simulink model "particle_sim"  (Simulink 8.7)
settings: Solver=ode3  StartTime=0.0  StopTime=inf  RelTol=1e-3
undefined symbols (not defined in the file or in its folder): ProperlyScaledOppositeMover
settings Model: Creator=KAMAK  LastModifiedBy=rcooper
settings DataIOCC: SignalLoggingSaveFormat=ModelDataLogs
settings OptimizationCC: ExpressionDepthLimit=2147483647
settings DebuggingCC: SolverPrmCheckMsg=warning  FcnCallInpInsideContextMsg=UseLocalSettings  StateNameClashWarn=warning
settings GRTTargetCC: CombineOutputUpdateFcns=off  GRTInterface=on

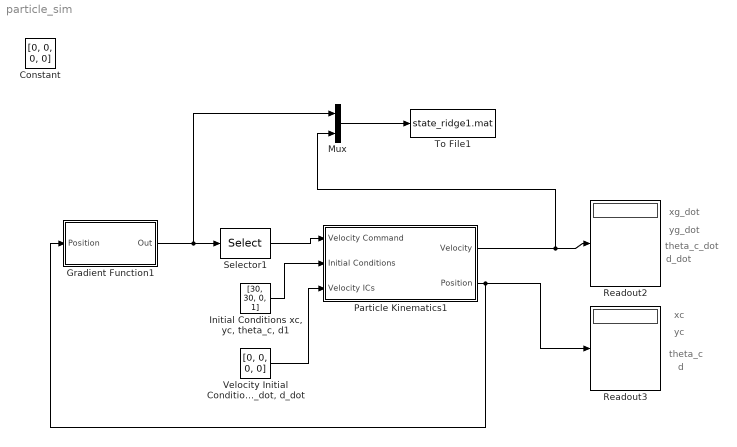
== system particle_sim ==
  note: xg_dot
  note: yg_dot
  note: theta_c_dot
  note: d_dot
  note: xc
  note: yc
  note: theta_c
  note: d
  Gradient Function1 : Subsystem
  "Initial Conditions xc, yc, theta_c, d1" : Constant  Value=[30, 30, 0, 1]  OutDataTypeStr=double
  Mux : Mux  Inputs=2
  Particle Kinematics1 : Subsystem
  Readout2 : Display
  Readout3 : Display
  Selector1 : Selector  InputPortWidth=24  IndexOptions=Index vector (dialog)  Indices=[1 2 3 4]  OutputSizes=1
  To File1 : ToFile  Filename=state_ridge1.mat  MatrixName=data  SaveFormat=Timeseries
  "Velocity Initial Conditions xg_dot, yg_dot, theta_c_dot, d_dot" : Constant  Value=[0, 0, 0, 0]
  Constant : Constant  IOType=siggen  Value=[0, 0, 0, 0]  VectorParams1D=off
  wires:
  "Initial Conditions xc, yc, theta_c, d1"/1 -> Particle Kinematics1/2(Initial Conditions)
  Gradient Function1/1(Out) -> Mux/1, Selector1/1
  Particle Kinematics1/2(Position) -> Gradient Function1/1(Position), Readout3/1
  Particle Kinematics1/1(Velocity) -> Mux/2, Readout2/1
  Selector1/1 -> Particle Kinematics1/1(Velocity Command)
  "Velocity Initial Conditions xg_dot, yg_dot, theta_c_dot, d_dot"/1 -> Particle Kinematics1/3(Velocity ICs)
  Mux/1 -> To File1/1

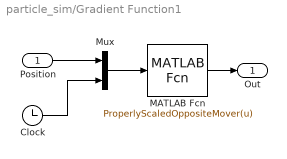
== system particle_sim/Gradient Function1 ==
  Position : Inport
  Clock : Clock
  MATLAB Fcn : MATLABFcn  MATLABFcn=ProperlyScaledOppositeMover(u)  OutputDimensions=24  Output1D=off
  Mux : Mux  Inputs=2
  Out : Outport
  wires:
  MATLAB Fcn/1 -> Out/1
  Clock/1 -> Mux/2
  Position/1 -> Mux/1
  Mux/1 -> MATLAB Fcn/1

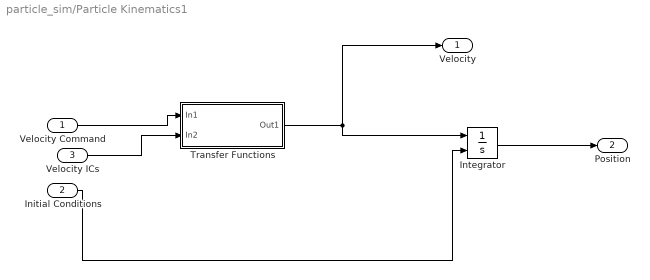
== system particle_sim/Particle Kinematics1 ==
  Velocity Command : Inport
  Initial Conditions : Inport  Port=2
  Velocity ICs : Inport  Port=3
  Integrator : Integrator  InitialConditionSource=external
  Transfer Functions : Subsystem
  Velocity : Outport
  Position : Outport  Port=2
  wires:
  Integrator/1 -> Position/1
  Initial Conditions/1 -> Integrator/2
  Transfer Functions/1(Out1) -> Velocity/1, Integrator/1
  Velocity Command/1 -> Transfer Functions/1(In1)
  Velocity ICs/1 -> Transfer Functions/2(In2)

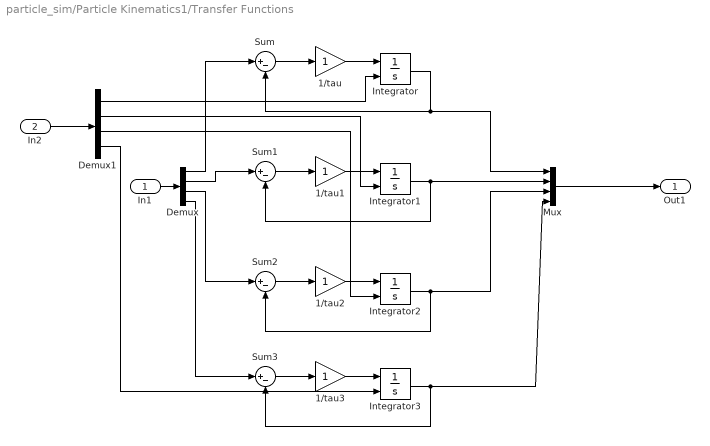
== system particle_sim/Particle Kinematics1/Transfer Functions ==
  In1 : Inport
  In2 : Inport  Port=2
  1/tau{,1..3} (4 alike) : Gain
  Demux : Demux
  Demux1 : Demux
  Integrator{,1..3} (4 alike) : Integrator  InitialConditionSource=external
  Mux : Mux
  Sum{,1..3} (4 alike) : Sum  Inputs=|+-
  Out1 : Outport
  wires:
  In1/1 -> Demux/1
  Demux/1 -> Sum/1
  Mux/1 -> Out1/1
  Sum/1 -> 1/tau/1
  1/tau/1 -> Integrator/1
  Integrator/1 -> Mux/1, Sum/2
  Sum1/1 -> 1/tau1/1
  1/tau1/1 -> Integrator1/1
  Integrator1/1 -> Sum1/2, Mux/2
  Demux/2 -> Sum1/1
  Demux/3 -> Sum2/1
  Sum2/1 -> 1/tau2/1
  1/tau2/1 -> Integrator2/1
  Integrator2/1 -> Sum2/2, Mux/3
  Sum3/1 -> 1/tau3/1
  1/tau3/1 -> Integrator3/1
  Integrator3/1 -> Sum3/2, Mux/4
  Demux/4 -> Sum3/1
  Demux1/1 -> Integrator/2
  Demux1/2 -> Integrator1/2
  Demux1/3 -> Integrator2/2
  Demux1/4 -> Integrator3/2
  In2/1 -> Demux1/1
